simulink model "cssm_task"  (Simulink 7.4)
libraries: modellib x2, mathlib x2, genlib x1, arclib x1
settings Model: Creator=pbalda  LastModifiedBy=pbalda  ExtModeTrigMode=oneshot  ExtModeArmWhenConnect=off

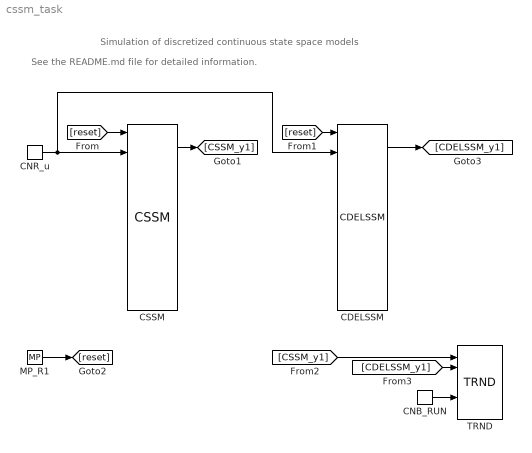
== system cssm_task ==
  note: See the README.md file for detailed information.
  note: Simulation of discretized continuous state space models
  CDELSSM : modellib/CDELSSM  SystemSampleTime=-1  UD=off  del=1.5  is=2  eps=1.0e-15  Ac=[-0.36 -1.24 -0.18; 1 0 0; 0 1 0]  Bc=[0.5; 0; 0]  Cc=[0.12 0.48 0.36]  Dc=[0]  x0=[0; 0; 0]
  CNB_RUN : mathlib/CNB  YCN=on
  CNR_u : mathlib/CNR  SystemSampleTime=-1  ycn=0
  CSSM : modellib/CSSM  SystemSampleTime=-1  UD=off  is=2  eps=1.0e-15  Ac="[-0.36  -1.24  -0.18; 1 0 0; 0 1  0]"  Bc=[0.5; 0; 0]  Cc=[0.12 0.48 0.36]  Dc=[0]  x0=[0; 0; 0]
  MP_R1 : genlib/MP  pwidth=0.001  BSTATE=off  RPTF=off
  TRND : arclib/TRND  n=2  l=200  btype=8: Double  ptype1=1: Store  ptype2=1: Store  ptype3=1: Store  ptype4=1: Store  pfac=1  afac=0  arc=0  id=1  Title=Trend Title  timesrc=1
  wires:
  CDELSSM/2 -> [CDELSSM_y1]
  CNB_RUN/1 -> TRND/5
  CNR_u/1 -> CDELSSM/3, CSSM/3
  CSSM/2 -> [CSSM_y1]
  [reset] -> CSSM/1
  [reset] -> CDELSSM/1
  [CSSM_y1] -> TRND/1
  [CDELSSM_y1] -> TRND/2
  MP_R1/1 -> [reset]
